simulink model "RampSpeed"  (Simulink 7.4)
settings: Solver=ode45  StartTime=0.0  StopTime=60  RelTol=1e-3
values from neighbouring files (symbols this model uses):
  speed = speed1(:,i)    [VGait_Input_Signals.m]
libraries: simulink x1
settings Model: Creator=Sandy  LastModifiedBy=Sandy

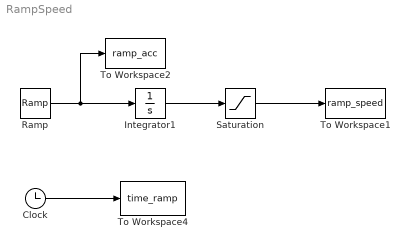
== system RampSpeed ==
  Clock : Clock
      settings: Decimation=10
  Integrator1 : Integrator
  Ramp : simulink/Sources/Ramp  SystemSampleTime=-1  slope=0.25  start=0  X0=0
  Saturation : Saturate  UpperLimit=speed  LowerLimit=0  OutDataType=fixdt(1, 16)  OutScaling=2^0
  To Workspace1 : ToWorkspace  VariableName=ramp_speed  SampleTime=0.0033  SaveFormat=Array
  To Workspace2 : ToWorkspace  VariableName=ramp_acc  SampleTime=0.0033  SaveFormat=Array
  To Workspace4 : ToWorkspace  VariableName=time_ramp  SampleTime=0.0033  SaveFormat=Array
  wires:
  Ramp/1 -> Integrator1/1, To Workspace2/1
  Saturation/1 -> To Workspace1/1
  Integrator1/1 -> Saturation/1
  Clock/1 -> To Workspace4/1
